simulink subsystem "Bluetooth_Velocidad"  (R2024b)
settings: Solver=VariableStepAuto  StartTime=0.0  StopTime=10.0  RelTol=1e-3
settings Model: Creator=Chenfu  LastModifiedBy=Chenfu

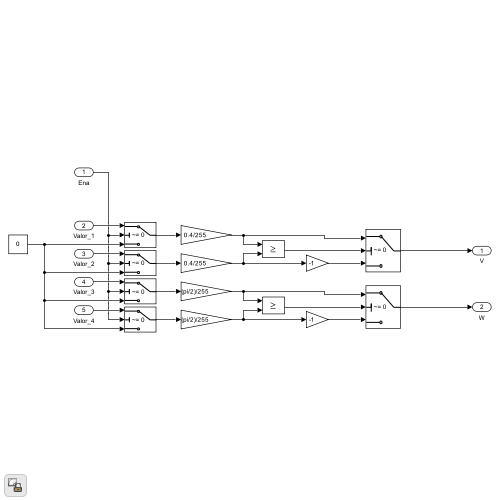
[thumbnail: Simulink's stored preview of the top-level diagram]
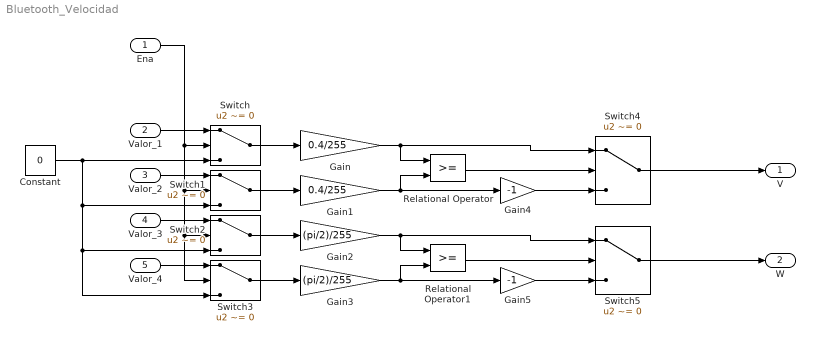
== system Bluetooth_Velocidad ==
  Ena : Inport
  Valor_1 : Inport  Port=2
  Valor_2 : Inport  Port=3
  Valor_3 : Inport  Port=4
  Valor_4 : Inport  Port=5
  Constant : Constant  Value=0  OutDataTypeStr='uint8'
  Gain : Gain  Gain=0.4/255  OutDataTypeStr='double'
  Gain1 : Gain  Gain=0.4/255  OutDataTypeStr='double'
  Gain2 : Gain  Gain=(pi/2)/255  OutDataTypeStr='double'
  Gain3 : Gain  Gain=(pi/2)/255  OutDataTypeStr='double'
  Gain4 : Gain  Gain=-1  OutDataTypeStr='double'
  Gain5 : Gain  Gain=-1  OutDataTypeStr='double'
  Relational Operator : RelationalOperator  OutDataTypeStr=boolean  RndMeth=Simplest  InputSameDT=off
  Relational Operator1 : RelationalOperator  OutDataTypeStr=boolean  RndMeth=Simplest  InputSameDT=off
  Switch{,1..5} (6 alike) : Switch  Criteria=u2 ~= 0  SaturateOnIntegerOverflow=off  InputSameDT=off
  V : Outport
  W : Outport  Port=2
  wires:
  Switch/1 -> Gain/1
  Switch1/1 -> Gain1/1
  Switch2/1 -> Gain2/1
  Switch3/1 -> Gain3/1
  Valor_4/1 -> Switch3/1
  Valor_3/1 -> Switch2/1
  Valor_2/1 -> Switch1/1
  Constant/1 -> Switch/3, Switch2/3, Switch3/3, Switch1/3
  Ena/1 -> Switch2/2, Switch3/2, Switch1/2, Switch/2
  Valor_1/1 -> Switch/1
  Gain/1 -> Relational Operator/1, Switch4/1
  Gain1/1 -> Gain4/1, Relational Operator/2
  Relational Operator/1 -> Switch4/2
  Switch4/1 -> V/1
  Gain4/1 -> Switch4/3
  Gain3/1 -> Gain5/1, Relational Operator1/2
  Gain2/1 -> Relational Operator1/1, Switch5/1
  Gain5/1 -> Switch5/3
  Switch5/1 -> W/1
  Relational Operator1/1 -> Switch5/2
